simulink library "HelicopterBlockset"  (Simulink 5.0)
values from neighbouring files (symbols this model uses):
  alt_err_limit = 20    [DESIGNOR.M]    (also in HELICOPT.MAT)
  body_inertia = [0.8  0  0; 0  5  0; 0  0  5]    [HELICOPT.MAT]    (also in MODELPAR.M = body_mass *      [body_radius^2/2 0 0; 0 body_length^2/2 0; )
  body_mass = 10    [HELICOPT.MAT]    (also in MODELPAR.M)
  Cd = 0.1    [HELICOPT.MAT]    (also in MODELPAR.M)
  Cp = 0.10    (= 0.1)    [DESIGNOR.M]    (also in HELICOPT.MAT)
  Cq = 0.15    [DESIGNOR.M]    (also in HELICOPT.MAT)
  dt = 0.01    [HELICOPT.MAT]    (also in MODELPAR.M)
  Kd = 5    [DESIGNOR.M]    (also in HELICOPT.MAT)
  Kp = 0.8    [DESIGNOR.M]    (also in HELICOPT.MAT)
  mr_angle_ic = 90    [HELICOPT.MAT]    (also in MODELPAR.M)
  mr_inertia = [3.125e-05  0  0; 0  0.05  0; 0  0  0.05]    [HELICOPT.MAT]    (also in MODELPAR.M = mr_mass *      [mr_radius^2/2 0 0; 0 mr_length^2/2 0; 0 0 mr)
  mr_mass = 0.1    [HELICOPT.MAT]    (also in MODELPAR.M)
  mr_vel = -7161.97243914    [HELICOPT.MAT]    (also in MODELPAR.M)
  N = Nu + K*Nx    [SSDESIGN.M]
  N_p = 36.4154159163    [HELICOPT.MAT]
  N_r = -5.86917812224    [HELICOPT.MAT]
  N_v = 5.28688842277    [HELICOPT.MAT]
  N_y = -0.0302858280261    [HELICOPT.MAT]
  ssobsctrl_p =     [HELICOPT.MAT]
  ssobsctrl_r =     [HELICOPT.MAT]
  ssobsctrl_v =     [HELICOPT.MAT]
  ssobsctrl_y =     [HELICOPT.MAT]
  tau = 0.8    [DESIGNOR.M]    (also in HELICOPT.MAT)
  tilt_limit = 5    [DESIGNOR.M]    (also in HELICOPT.MAT)
  tr_inertia = [1.125e-06  0  0; 0  0.0008  0; 0  0  0.0008]    [HELICOPT.MAT]    (also in MODELPAR.M = tr_mass *      [tr_radius^2/2 0 0; 0 tr_length^2/2 0; 0 0 tr)
  tr_mass = 0.01    [HELICOPT.MAT]    (also in MODELPAR.M)
  tr_vel = 14323.9448783    [HELICOPT.MAT]    (also in MODELPAR.M)
  trim_lift_force = -99.1791    [HELICOPT.MAT]    (also in MODELPAR.M = -(body_mass + mr_mass + tr_mass) * gravity_vector(3))
  trim_pitch_mom = -0.04905    [HELICOPT.MAT]    (also in MODELPAR.M = (mr_mass*(mr_position(1) - body_position_ic(1)) +      tr_ma)
  waypoint = [-100 -100 0 0 -100 -100 -200 -200 -100 -100 -200 -200 ... (84 elements, 14x6)]    [HELICOPT.MAT]    (also in MODELPAR.M = [      100,   0,  25,  0,  0,  0;      100, 100,  25,  0,  0)
undefined symbols (not defined in the file or in its folder): Ad, Bd, Dd, dend, icd, numd
libraries: fixpt_lib_4 x19, mblibv1 x18, simulink x3, discretizing x1
settings Model: LastModifiedBy=Jim

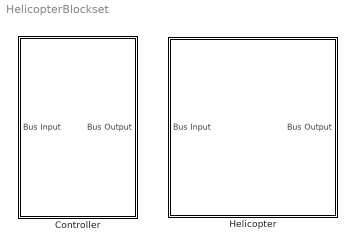
== system HelicopterBlockset ==
  Controller : Subsystem  TreatAsAtomicUnit=on
  Helicopter : Subsystem

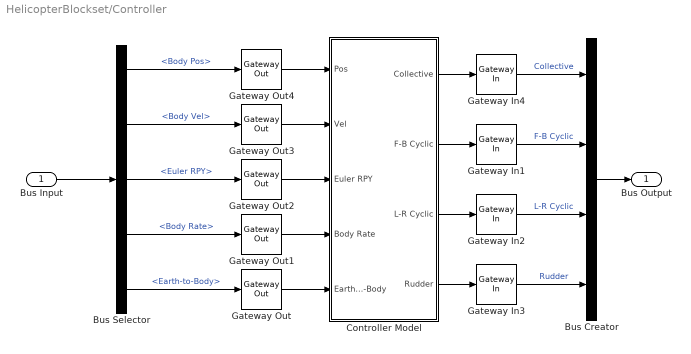
== system HelicopterBlockset/Controller ==
  Bus Input : Inport
  Bus Creator : BusCreator
  Bus Selector : BusSelector  OutputSignals=Body Pos,Body Vel,Euler RPY,Body Rate,Earth-to-Body
  Controller Model : Subsystem
  Gateway In{1..4} (4 alike) : fixpt_lib_4/Data Type/Gateway In  InRealWorld=Real World Value  OutputDataTypeScalingMode=Specify via dialog  OutDataType=sfix(16)  OutScaling=2^-8  RndMeth=Nearest  DoSatur=on
  Gateway Out{,1..4} (5 alike) : fixpt_lib_4/Data Type/Gateway Out  OutRealWorld=Real World Value  OutBuiltInType=double  RndMeth=Nearest  DoSatur=off
  Bus Output : Outport
  wires:
  Gateway In3/1 -> Bus Creator/4  "Rudder"
  Gateway In2/1 -> Bus Creator/3  "L-R Cyclic"
  Gateway In1/1 -> Bus Creator/2  "F-B Cyclic"
  Gateway In4/1 -> Bus Creator/1  "Collective"
  Gateway Out4/1 -> Controller Model/1(Pos)
  Gateway Out3/1 -> Controller Model/2(Vel)
  Gateway Out2/1 -> Controller Model/3(Euler RPY)
  Gateway Out1/1 -> Controller Model/4(Body Rate)
  Gateway Out/1 -> Controller Model/5(Earth-to-Body)
  Bus Input/1 -> Bus Selector/1
  Bus Creator/1 -> Bus Output/1
  Controller Model/4(Rudder) -> Gateway In3/1
  Bus Selector/2 -> Gateway Out3/1  "<Body Vel>"
  Controller Model/3(L-R Cyclic) -> Gateway In2/1
  Bus Selector/5 -> Gateway Out/1  "<Earth-to-Body>"
  Controller Model/2(F-B Cyclic) -> Gateway In1/1
  Controller Model/1(Collective) -> Gateway In4/1
  Bus Selector/4 -> Gateway Out1/1  "<Body Rate>"
  Bus Selector/3 -> Gateway Out2/1  "<Euler RPY>"
  Bus Selector/1 -> Gateway Out4/1  "<Body Pos>"

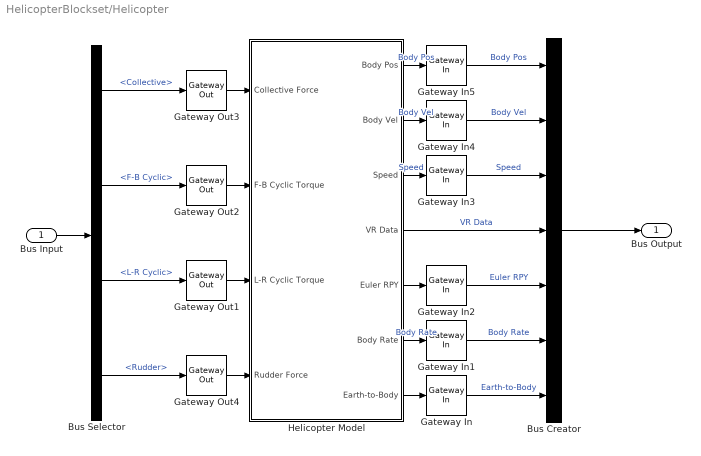
== system HelicopterBlockset/Helicopter ==
  Bus Input : Inport
  Bus Creator : BusCreator  Inputs=7
  Bus Selector : BusSelector  OutputSignals=Collective,F-B Cyclic,L-R Cyclic,Rudder
  Gateway In : fixpt_lib_4/Data Type/Gateway In  InRealWorld=Real World Value  OutputDataTypeScalingMode=Specify via dialog  OutDataType=sfix(8)  OutScaling=2^-7  RndMeth=Nearest  DoSatur=on
  Gateway In1 : fixpt_lib_4/Data Type/Gateway In  InRealWorld=Real World Value  OutputDataTypeScalingMode=Specify via dialog  OutDataType=sfix(16)  OutScaling=2^-7  RndMeth=Nearest  DoSatur=on
  Gateway In2 : fixpt_lib_4/Data Type/Gateway In  InRealWorld=Real World Value  OutputDataTypeScalingMode=Specify via dialog  OutDataType=sfix(16)  OutScaling=2^-7  RndMeth=Nearest  DoSatur=on
  Gateway In3 : fixpt_lib_4/Data Type/Gateway In  InRealWorld=Real World Value  OutputDataTypeScalingMode=Specify via dialog  OutDataType=sfix(16)  OutScaling=2^-8  RndMeth=Nearest  DoSatur=on
  Gateway In4 : fixpt_lib_4/Data Type/Gateway In  InRealWorld=Real World Value  OutputDataTypeScalingMode=Specify via dialog  OutDataType=sfix(16)  OutScaling=2^-8  RndMeth=Nearest  DoSatur=on
  Gateway In5 : fixpt_lib_4/Data Type/Gateway In  InRealWorld=Real World Value  OutputDataTypeScalingMode=Specify via dialog  OutDataType=sfix(32)  OutScaling=2^-4  RndMeth=Nearest  DoSatur=on
  Gateway Out{1..4} (4 alike) : fixpt_lib_4/Data Type/Gateway Out  OutRealWorld=Real World Value  OutBuiltInType=double  RndMeth=Nearest  DoSatur=off
  Helicopter Model : Subsystem
  Bus Output : Outport
  wires:
  Gateway Out3/1 -> Helicopter Model/1(Collective Force)
  Gateway Out2/1 -> Helicopter Model/2(F-B Cyclic Torque)
  Gateway Out1/1 -> Helicopter Model/3(L-R Cyclic Torque)
  Gateway Out4/1 -> Helicopter Model/4(Rudder Force)
  Gateway In5/1 -> Bus Creator/1  "Body Pos"
  Gateway In4/1 -> Bus Creator/2  "Body Vel"
  Gateway In3/1 -> Bus Creator/3  "Speed"
  Gateway In2/1 -> Bus Creator/5  "Euler RPY"
  Gateway In1/1 -> Bus Creator/6  "Body Rate"
  Gateway In/1 -> Bus Creator/7  "Earth-to-Body"
  Bus Creator/1 -> Bus Output/1
  Bus Input/1 -> Bus Selector/1
  Helicopter Model/7(Earth-to-Body) -> Gateway In/1
  Bus Selector/4 -> Gateway Out4/1  "<Rudder>"
  Helicopter Model/6(Body Rate) -> Gateway In1/1  "Body Rate"
  Helicopter Model/5(Euler RPY) -> Gateway In2/1
  Helicopter Model/4(VR Data) -> Bus Creator/4  "VR Data"
  Helicopter Model/3(Speed) -> Gateway In3/1  "Speed"
  Helicopter Model/2(Body Vel) -> Gateway In4/1  "Body Vel"
  Bus Selector/3 -> Gateway Out1/1  "<L-R Cyclic>"
  Helicopter Model/1(Body Pos) -> Gateway In5/1  "Body Pos"
  Bus Selector/2 -> Gateway Out2/1  "<F-B Cyclic>"
  Bus Selector/1 -> Gateway Out3/1  "<Collective>"

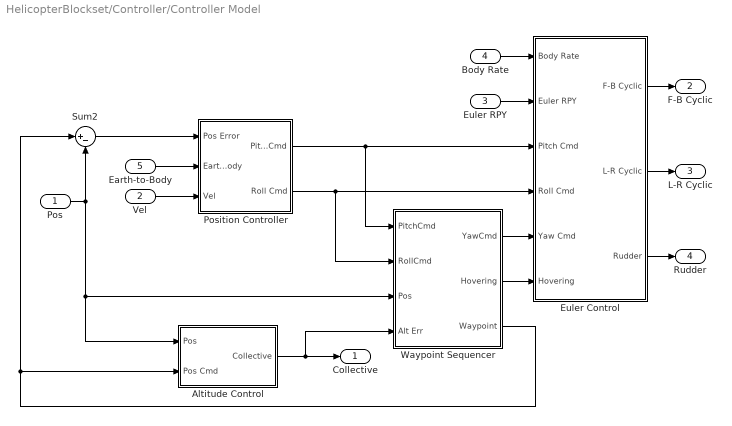
== system HelicopterBlockset/Controller/Controller Model ==
  Pos : Inport
  Vel : Inport  Port=2
  Euler RPY : Inport  Port=3
  Body Rate : Inport  Port=4
  Earth-to-Body : Inport  Port=5
  Altitude Control : Subsystem
  Euler Control : Subsystem
  Position Controller : Subsystem
  Sum2 : Sum  Inputs=|+-  SaturateOnIntegerOverflow=on
  Waypoint Sequencer : Subsystem
  Collective : Outport
  F-B Cyclic : Outport  Port=2
  L-R Cyclic : Outport  Port=3
  Rudder : Outport  Port=4
  wires:
  Waypoint Sequencer/2(Hovering) -> Euler Control/6(Hovering)
  Earth-to-Body/1 -> Position Controller/2(Earth-to-Body)
  Euler Control/3(Rudder) -> Rudder/1
  Euler Control/2(L-R Cyclic) -> L-R Cyclic/1
  Euler Control/1(F-B Cyclic) -> F-B Cyclic/1
  Euler RPY/1 -> Euler Control/2(Euler RPY)
  Body Rate/1 -> Euler Control/1(Body Rate)
  Altitude Control/1(Collective) -> Collective/1, Waypoint Sequencer/4(Alt Err)
  Vel/1 -> Position Controller/3(Vel)
  Waypoint Sequencer/1(YawCmd) -> Euler Control/5(Yaw Cmd)
  Pos/1 -> Sum2/2, Waypoint Sequencer/3(Pos), Altitude Control/1(Pos)
  Sum2/1 -> Position Controller/1(Pos Error)
  Position Controller/2(Roll Cmd) -> Euler Control/4(Roll Cmd), Waypoint Sequencer/2(RollCmd)
  Position Controller/1(Pitch Cmd) -> Euler Control/3(Pitch Cmd), Waypoint Sequencer/1(PitchCmd)
  Waypoint Sequencer/3(Waypoint) -> Altitude Control/2(Pos Cmd), Sum2/1

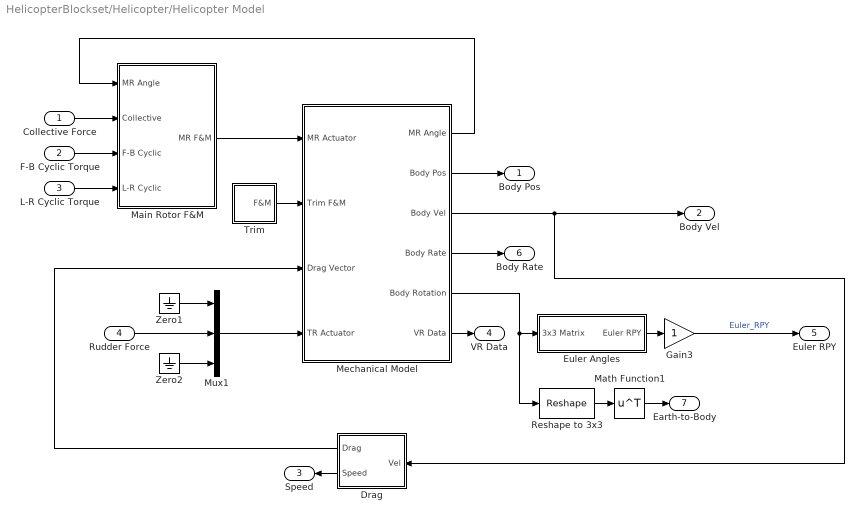
== system HelicopterBlockset/Helicopter/Helicopter Model ==
  Collective Force : Inport
  F-B Cyclic Torque : Inport  Port=2
  L-R Cyclic Torque : Inport  Port=3
  Rudder Force : Inport  Port=4
  Drag : Subsystem  Orientation=left
  Euler Angles : Subsystem
  Gain3 : Gain  SaturateOnIntegerOverflow=on
  Main Rotor F&M : Subsystem
  Math Function1 : Math  Operator=transpose
  Mechanical Model : Subsystem
  Mux1 : Mux  Inputs=3
  Reshape to 3x3 : simulink/Math Operations/Reshape  OutputDimensionality=Customize  OutputDimensions=[3,3]
  Trim : Subsystem
  Zero1 : Ground
  Zero2 : Ground
  Body Pos : Outport
  Body Vel : Outport  Port=2
  Speed : Outport  Orientation=left  Port=3
  VR Data : Outport  Port=4
  Euler RPY : Outport  Port=5  InitialOutput=0
  Body Rate : Outport  Port=6
  Earth-to-Body : Outport  Port=7  InitialOutput=0
  wires:
  Gain3/1 -> Euler RPY/1  "Euler_RPY"
  Drag/2(Speed) -> Speed/1
  Mechanical Model/6(VR Data) -> VR Data/1
  Mechanical Model/2(Body Pos) -> Body Pos/1
  Mechanical Model/3(Body Vel) -> Body Vel/1, Drag/1(Vel)
  Main Rotor F&M/1(MR F&M) -> Mechanical Model/1(MR Actuator)
  Mux1/1 -> Mechanical Model/4(TR Actuator)
  Zero1/1 -> Mux1/1
  Euler Angles/1(Euler RPY) -> Gain3/1
  L-R Cyclic Torque/1 -> Main Rotor F&M/4(L-R Cyclic)
  F-B Cyclic Torque/1 -> Main Rotor F&M/3(F-B Cyclic)
  Rudder Force/1 -> Mux1/2
  Collective Force/1 -> Main Rotor F&M/2(Collective)
  Trim/1(F&M) -> Mechanical Model/2(Trim F&M)
  Mechanical Model/4(Body Rate) -> Body Rate/1
  Mechanical Model/5(Body Rotation) -> Euler Angles/1(3x3 Matrix), Reshape to 3x3/1
  Reshape to 3x3/1 -> Math Function1/1
  Math Function1/1 -> Earth-to-Body/1
  Mechanical Model/1(MR Angle) -> Main Rotor F&M/1(MR Angle)
  Zero2/1 -> Mux1/3
  Drag/1(Drag) -> Mechanical Model/3(Drag Vector)

== system HelicopterBlockset/Controller/Controller Model/Altitude Control ==
  Pos : Inport
  Pos Cmd : Inport  Port=2
  Alt Limit : Saturate  UpperLimit=alt_err_limit  LowerLimit=-alt_err_limit
  Altitude Controller : Subsystem
  Demux1 : Demux  Outputs=3
  Demux2 : Demux  Outputs=3
  Terminator{2..3,5..6} (4 alike) : Terminator
  Collective : Outport
  wires:
  Alt Limit/1 -> Collective/1
  Pos Cmd/1 -> Demux1/1
  Pos/1 -> Demux2/1
  Altitude Controller/1(u) -> Alt Limit/1
  Demux2/2 -> Terminator6/1
  Demux2/1 -> Terminator5/1
  Demux2/3 -> Altitude Controller/2(y)
  Demux1/3 -> Altitude Controller/1(r)
  Demux1/1 -> Terminator3/1
  Demux1/2 -> Terminator2/1

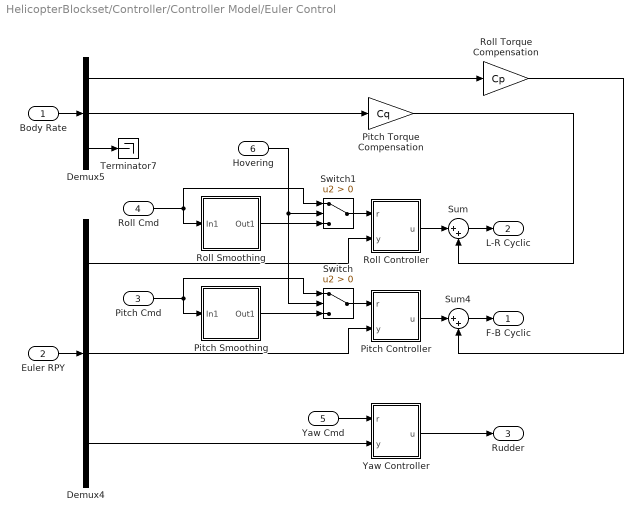
== system HelicopterBlockset/Controller/Controller Model/Euler Control ==
  Body Rate : Inport
  Euler RPY : Inport  Port=2
  Pitch Cmd : Inport  Port=3
  Roll Cmd : Inport  Port=4
  Yaw Cmd : Inport  Port=5
  Hovering : Inport  Port=6
  Demux4 : Demux  Outputs=3
  Demux5 : Demux  Outputs=3
  Pitch Controller : Subsystem
  Pitch Smoothing : Subsystem  mask(DiscretizedTransferFcn){Numerator=[1], Denominator=[tau 1], AbsTol=auto, SampleTime=dt, method=foh, Wc=1}
      mask prompts: Numerator "Numerator (enter in s-domain:)"; Denominator "Denominator (enter in s-domain:)"; AbsTol "Absolute tolerance:"; SampleTime "Sample time:"; Wc "Critical Frequency (Hz):"
      mask help: Continuous mask uses c2d to transform parameters onto the Discrete Transfer function block inside.
      mask init:
      | st=SampleTime;
      | if length(st)>1
      |     st=SampleTime(1);
      | end
      | if(st>0)
      |     [numd,dend] = sldiscutil('disctransferfcn',{st,method,Wc,Numerator,Denominator});
      | end	
      | s = get_param(gcb,'maskvalues');
      | nums = s{1};
      | dens = s{2};
      | %numc = eval(nums);
      | %denc = eval(dens);
      | sldiscutil('inittfmask', st);
      | if(st==0)
      | set_param([gcb '/Transfer Fcn'], 'AbsoluteTolerance', AbsTol);
      | end
      mask StyleString: edit,edit,edit,edit,popup(zoh|foh|tustin|prewarp|matched),edit
      mask CallbackString: ||||hidecrit|
      mask Display:
      | dpoly(nums,dens)
      | text( 0.5, 1.0, method, 'verticalAlignment','top')
  Pitch Torque Compensation : Gain  Gain=Cq  SaturateOnIntegerOverflow=on
  Roll Controller : Subsystem
  Roll Smoothing : Subsystem  mask(DiscretizedTransferFcn){Numerator=[1], Denominator=[tau 1], AbsTol=auto, SampleTime=dt, method=foh, Wc=1}
      mask prompts: Numerator "Numerator (enter in s-domain:)"; Denominator "Denominator (enter in s-domain:)"; AbsTol "Absolute tolerance:"; SampleTime "Sample time:"; Wc "Critical Frequency (Hz):"
      mask help: Continuous mask uses c2d to transform parameters onto the Discrete Transfer function block inside.
      mask init: same as HelicopterBlockset/Controller/Controller Model/Euler Control/Pitch Smoothing
      mask StyleString: edit,edit,edit,edit,popup(zoh|foh|tustin|prewarp|matched),edit
      mask CallbackString: ||||hidecrit|
      mask Display:
      | dpoly(nums,dens)
      | text( 0.5, 1.0, method, 'verticalAlignment','top')
  Roll Torque Compensation : Gain  Gain=Cp  SaturateOnIntegerOverflow=on
  Sum : Sum  Inputs=|++  SaturateOnIntegerOverflow=on
  Sum4 : Sum  Inputs=|++  SaturateOnIntegerOverflow=on
  Switch : Switch  Criteria=u2 > Threshold  SaturateOnIntegerOverflow=on
  Switch1 : Switch  Criteria=u2 > Threshold  SaturateOnIntegerOverflow=on
  Terminator7 : Terminator
  Yaw Controller : Subsystem
  F-B Cyclic : Outport
  L-R Cyclic : Outport  Port=2
  Rudder : Outport  Port=3
  wires:
  Roll Cmd/1 -> Switch1/1, Roll Smoothing/1(In1)
  Roll Smoothing/1(Out1) -> Switch1/3
  Pitch Smoothing/1(Out1) -> Switch/3
  Hovering/1 -> Switch/2, Switch1/2
  Switch1/1 -> Roll Controller/1(r)
  Pitch Cmd/1 -> Switch/1, Pitch Smoothing/1(In1)
  Switch/1 -> Pitch Controller/1(r)
  Yaw Controller/1(u) -> Rudder/1
  Yaw Cmd/1 -> Yaw Controller/1(r)
  Sum/1 -> L-R Cyclic/1
  Sum4/1 -> F-B Cyclic/1
  Euler RPY/1 -> Demux4/1
  Body Rate/1 -> Demux5/1
  Roll Controller/1(u) -> Sum/1
  Pitch Controller/1(u) -> Sum4/1
  Roll Torque Compensation/1 -> Sum4/2
  Demux5/1 -> Roll Torque Compensation/1
  Pitch Torque Compensation/1 -> Sum/2
  Demux5/2 -> Pitch Torque Compensation/1
  Demux5/3 -> Terminator7/1
  Demux4/3 -> Yaw Controller/2(y)
  Demux4/1 -> Roll Controller/2(y)
  Demux4/2 -> Pitch Controller/2(y)

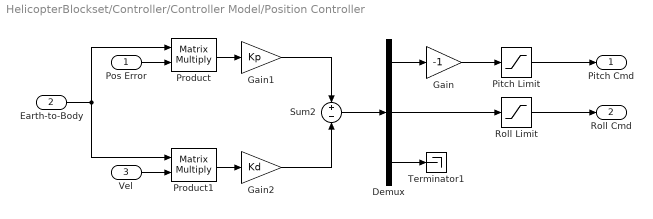
== system HelicopterBlockset/Controller/Controller Model/Position Controller ==
  Pos Error : Inport
  Earth-to-Body : Inport  Port=2
  Vel : Inport  Port=3
  Demux : Demux  Outputs=3
  Gain : Gain  Gain=-1  SaturateOnIntegerOverflow=on
  Gain1 : Gain  Gain=Kp  SaturateOnIntegerOverflow=on
  Gain2 : Gain  Gain=Kd  SaturateOnIntegerOverflow=on
  Pitch Limit : Saturate  UpperLimit=tilt_limit  LowerLimit=-tilt_limit
  Product : Product  Multiplication=Matrix(*)  SaturateOnIntegerOverflow=on
  Product1 : Product  Multiplication=Matrix(*)  SaturateOnIntegerOverflow=on
  Roll Limit : Saturate  UpperLimit=tilt_limit  LowerLimit=-tilt_limit
  Sum2 : Sum  Inputs=+|-  SaturateOnIntegerOverflow=on
  Terminator1 : Terminator
  Pitch Cmd : Outport
  Roll Cmd : Outport  Port=2
  wires:
  Roll Limit/1 -> Roll Cmd/1
  Pitch Limit/1 -> Pitch Cmd/1
  Gain/1 -> Pitch Limit/1
  Demux/1 -> Gain/1
  Demux/2 -> Roll Limit/1
  Sum2/1 -> Demux/1
  Gain2/1 -> Sum2/2
  Gain1/1 -> Sum2/1
  Vel/1 -> Product1/2
  Pos Error/1 -> Product/2
  Product1/1 -> Gain2/1
  Earth-to-Body/1 -> Product/1, Product1/1
  Product/1 -> Gain1/1
  Demux/3 -> Terminator1/1

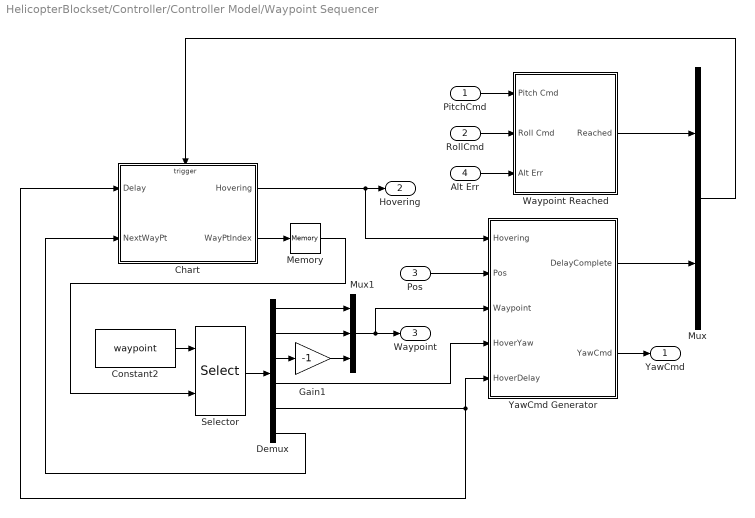
== system HelicopterBlockset/Controller/Controller Model/Waypoint Sequencer ==
  PitchCmd : Inport
  RollCmd : Inport  Port=2
  Pos : Inport  Port=3
  Alt Err : Inport  Port=4
  Chart : Stateflow chart
  Constant2 : Constant  Value=waypoint
  Demux : Demux  Outputs=6
  Gain1 : Gain  Gain=-1  SaturateOnIntegerOverflow=on
  Memory : Memory  X0=1
  Mux : Mux  Inputs=2
  Mux1 : Mux  Inputs=3
  Selector : Selector  InputType=Matrix  Elements=[1 3]  RowSrc=External  Columns=-1  InputPortWidth=3
  Waypoint Reached : Subsystem
  YawCmd Generator : Subsystem
  YawCmd : Outport
  Hovering : Outport  Port=2
  Waypoint : Outport  Port=3
  wires:
  Demux/6 -> Chart/2(NextWayPt)
  Chart/1(Hovering) -> Hovering/1, YawCmd Generator/1(Hovering)
  Gain1/1 -> Mux1/3
  Demux/3 -> Gain1/1
  Demux/2 -> Mux1/2
  Demux/1 -> Mux1/1
  Demux/4 -> YawCmd Generator/4(HoverYaw)
  Demux/5 -> Chart/1(Delay), YawCmd Generator/5(HoverDelay)
  YawCmd Generator/1(DelayComplete) -> Mux/2
  Memory/1 -> Selector/2
  YawCmd Generator/2(YawCmd) -> YawCmd/1
  Pos/1 -> YawCmd Generator/2(Pos)
  Chart/2(WayPtIndex) -> Memory/1
  Mux1/1 -> YawCmd Generator/3(Waypoint), Waypoint/1
  Mux/1 -> Chart/Trigger
  Waypoint Reached/1(Reached) -> Mux/1
  Constant2/1 -> Selector/1
  Selector/1 -> Demux/1
  Alt Err/1 -> Waypoint Reached/3(Alt Err)
  RollCmd/1 -> Waypoint Reached/2(Roll Cmd)
  PitchCmd/1 -> Waypoint Reached/1(Pitch Cmd)

== system HelicopterBlockset/Helicopter/Helicopter Model/Drag ==
  Vel : Inport
  Constant2 : Constant  Value=-Cd
  Dot Product : simulink/Math Operations/Dot Product
  Gain1 : Gain  SaturateOnIntegerOverflow=on
  Math Function : Math  Operator=sqrt
  Product2 : Product  Inputs=3  SaturateOnIntegerOverflow=on
  Drag : Outport
  Speed : Outport  Port=2
  wires:
  Gain1/1 -> Speed/1  "Speed"
  Dot Product/1 -> Math Function/1
  Math Function/1 -> Gain1/1, Product2/3
  Constant2/1 -> Product2/1
  Product2/1 -> Drag/1
  Vel/1 -> Dot Product/1, Dot Product/2, Product2/2

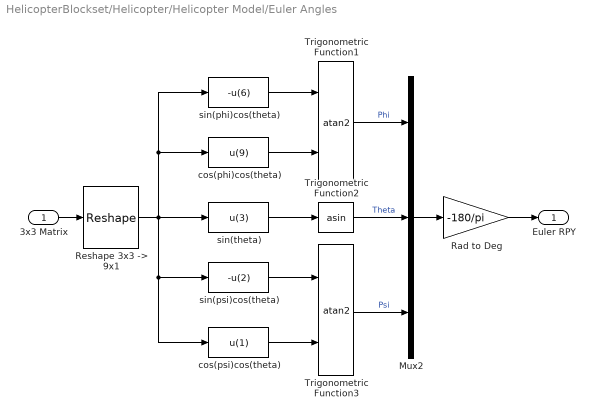
== system HelicopterBlockset/Helicopter/Helicopter Model/Euler Angles ==
  3x3 Matrix : Inport
  Mux2 : Mux  Inputs=3
  Rad to Deg : Gain  Gain=-180/pi  SaturateOnIntegerOverflow=on
  "Reshape 3x3 -> 9x1" : simulink/Math Operations/Reshape  OutputDimensionality=Column vector  OutputDimensions=[1,1]
  Trigonometric Function1 : Trigonometry  Operator=atan2
  Trigonometric Function2 : Trigonometry  Operator=asin
  Trigonometric Function3 : Trigonometry  Operator=atan2
  cos(phi)cos(theta) : Fcn  Expr=u(9)
  cos(psi)cos(theta) : Fcn  Expr=u(1)
  sin(phi)cos(theta) : Fcn  Expr=-u(6)
  sin(psi)cos(theta) : Fcn  Expr=-u(2)
  sin(theta) : Fcn  Expr=u(3)
  Euler RPY : Outport  InitialOutput=0
  wires:
  3x3 Matrix/1 -> "Reshape 3x3 -> 9x1"/1
  sin(theta)/1 -> Trigonometric Function2/1
  sin(phi)cos(theta)/1 -> Trigonometric Function1/1
  cos(phi)cos(theta)/1 -> Trigonometric Function1/2
  sin(psi)cos(theta)/1 -> Trigonometric Function3/1
  cos(psi)cos(theta)/1 -> Trigonometric Function3/2
  Trigonometric Function1/1 -> Mux2/1  "Phi"
  Trigonometric Function2/1 -> Mux2/2  "Theta"
  Trigonometric Function3/1 -> Mux2/3  "Psi"
  Mux2/1 -> Rad to Deg/1
  "Reshape 3x3 -> 9x1"/1 -> sin(theta)/1, sin(phi)cos(theta)/1, cos(phi)cos(theta)/1, sin(psi)cos(theta)/1, cos(psi)cos(theta)/1
  Rad to Deg/1 -> Euler RPY/1

== system HelicopterBlockset/Helicopter/Helicopter Model/Main Rotor F&M ==
  MR Angle : Inport
  Collective : Inport  Port=2
  F-B Cyclic : Inport  Port=3
  L-R Cyclic : Inport  Port=4
  Cosine of Blade Angle : Trigonometry  Operator=cos
  Mux : Mux  Inputs=6
  Product : Product  SaturateOnIntegerOverflow=on
  Product1 : Product  SaturateOnIntegerOverflow=on
  Sine of Blade Angle : Trigonometry
  Sum : Sum  Inputs=|++  SaturateOnIntegerOverflow=on
  Zero : Ground
  Zero1 : Ground
  MR F&M : Outport
  wires:
  MR Angle/1 -> Sine of Blade Angle/1, Cosine of Blade Angle/1
  Sine of Blade Angle/1 -> Product1/1
  Product1/1 -> Sum/2
  Product/1 -> Sum/1
  Cosine of Blade Angle/1 -> Product/1
  Sum/1 -> Mux/2
  Mux/1 -> MR F&M/1
  F-B Cyclic/1 -> Product/2
  L-R Cyclic/1 -> Product1/2
  Zero1/1 -> Mux/3, Mux/5, Mux/4
  Collective/1 -> Mux/6
  Zero/1 -> Mux/1

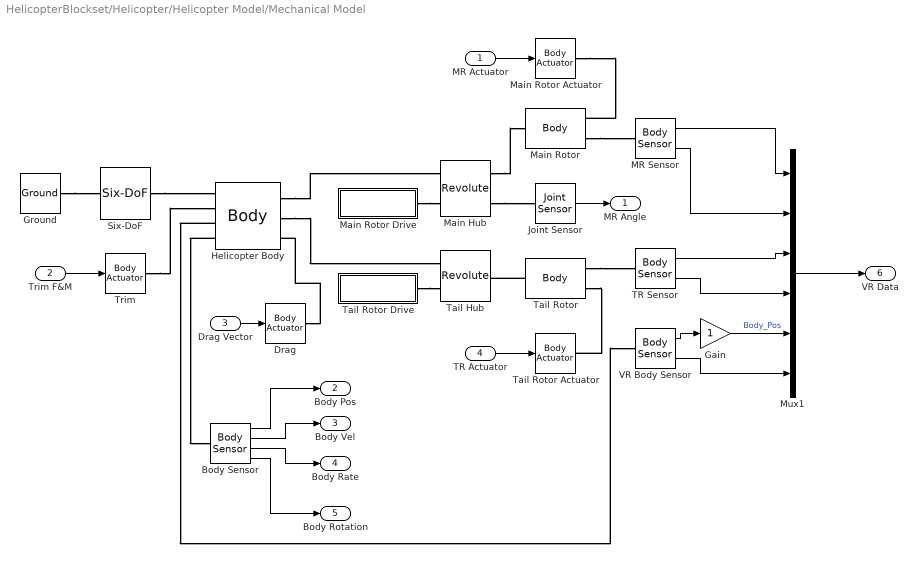
== system HelicopterBlockset/Helicopter/Helicopter Model/Mechanical Model ==
  MR Actuator : Inport
  Trim F&M : Inport  Port=2
  Drag Vector : Inport  Port=3
  TR Actuator : Inport  Port=4
  Body Sensor : mblibv1/Sensors &  Actuators/Body Sensor  Tag=__orphan__  PortType=blob  PhysicalDomain=Mechanical  Muxed=off  Pose=on  Angle=on  AngleUnits=deg  ArcVelocity=on  ArcVelocityUnits=deg/s  ArcAcceleration=off  ArcAccelerationUnits=deg/s^2  CoordPosition=on  CoordPositionUnits=m  Velocity=on  VelocityUnits=m/s  Acceleration=off  AccelerationUnits=m/s^2  Quaternion=on  QuaternionDT=off  QuaternionDDT=off  QuaternionUnits=off  OutputVector=[ 3 3 3 9 ]  IOID=sim_mech_taga8271b5312325fb6  ActiveIO=off  Width=18  DialogClass=MechanicalSensorBlock  ReferenceFrame=Absolute (World)
  Drag : mblibv1/Sensors &  Actuators/Body Actuator  Tag=__orphan__  PortType=blob  PhysicalDomain=Mechanical  ActuationStyle=Force  AngleUnits=deg  ArcVelocityUnits=deg/s  ArcAccelerationUnits=deg/s^2  CoordPositionUnits=m  VelocityUnits=m/s  AccelerationUnits=m/s^2  ForceUnits=N  TorqueUnits=N-m  IOID=sim_mech_tag546f64686babd5e8  ActiveIO=off  Width=3  DialogClass=MechanicalActuatorBlock  ReferenceFrame=Absolute (World)  Angle=off  CoordPosition=on  Force=on  Torque=off
  Gain : Gain  SaturateOnIntegerOverflow=on
  Ground : mblibv1/Bodies/Ground  Tag=__orphan__  PortType=workingframe  PhysicalDomain=Mechanical  DialogClass=GroundBlock  CoordPosition=ground_position  CoordPositionUnits=m  StateVectorMgrId=-1  MachineId=[0 0]
  Helicopter Body : mblibv1/Bodies/Body  PhysicalDomain=mechanical  SubClassName=Unknown  PortType=workingframe  LConnTagsString=CS1|CS4|CS6|CG  RConnTagsString=CS2|CS3|CS5  DialogClass=MechanicalBodyBlock  Mass=body_mass  MassUnits=kg  InertiaUnits=kg*m^2  Inertia=body_inertia  Shape=Cylinder  ShapeDims=[1 1]  ShapeUnits=m  ShapeUse=false  Density=1  DensityUnits=kg/m^3  DensityUse=false  CG=Left$CG$body_position_ic$WORLD$WORLD$m$body_orientation_ic$Euler Z-Y-X$deg$WORLD$true  WorkingFrames=Left$CS1$[0 0 0]$CG$CG$m$[0 0 0]$Euler Z-Y-X$deg$CG$true#Right$CS2$mr_position$CG$CG$m$mr_orientation$Euler Z-Y-X$deg$CG$true#Right$CS3$tr_position$CG$CG$m$tr_orientation$Euler Z-Y-X$deg$CG$true#Left$CS4$[0 0 0]$CG$CG$m$[0 0 0]$Euler Z-Y-X$deg$CG$true#Right$CS5$[0 0 0]$CG$CG$m$[0 0 0]$Euler Z-Y-X$deg$WORLD$true#Left$CS6$[0 0 0]$WORLD$WORLD$m$[0 0 0]$Euler Z-Y-X$deg$WORLD$true
  Joint Sensor : mblibv1/Sensors &  Actuators/Joint Sensor  Tag=__orphan__  PortType=blob  PhysicalDomain=Mechanical  Muxed=on  Pose=off  Angle=on  AngleUnits=rad  ArcVelocity=off  ArcVelocityUnits=deg/s  ArcAcceleration=off  ArcAccelerationUnits=deg/s^2  CoordPosition=on  CoordPositionUnits=m  Velocity=off  VelocityUnits=m/s  Acceleration=off  AccelerationUnits=m/s^2  Quaternion=on  QuaternionDT=off  QuaternionDDT=off  QuaternionUnits=off  OutputVector=[ 1 ]  IOID=sim_mech_tag96aebed2dbdd8e86  ActiveIO=off  Width=1  DialogClass=MechanicalSensorBlock  Primitive=R1  Force=off  ForceUnits=N  Torque=off  TorqueUnits=N-m  ReferenceFrame=Absolute (INERTIAL)  ReactionSensedSide=Base  ReactionReferenceFrame=Absolute (World)  ReactionForce=off  ReactionForceUnits=N  ReactionMoment=off  ReactionMomentUnits=N-m
  MR Sensor : mblibv1/Sensors &  Actuators/Body Sensor  Tag=__orphan__  PortType=blob  PhysicalDomain=Mechanical  Muxed=off  Pose=on  Angle=on  AngleUnits=deg  ArcVelocity=off  ArcVelocityUnits=deg/s  ArcAcceleration=off  ArcAccelerationUnits=deg/s^2  CoordPosition=on  CoordPositionUnits=m  Velocity=off  VelocityUnits=m/s  Acceleration=off  AccelerationUnits=m/s^2  Quaternion=on  QuaternionDT=off  QuaternionDDT=off  QuaternionUnits=off  OutputVector=[ 3 9 ]  IOID=sim_mech_tag28ea6e92d6f2dcb9  ActiveIO=off  Width=12  DialogClass=MechanicalSensorBlock  ReferenceFrame=Absolute (World)
  Main Hub : mblibv1/Joints/Revolute  PhysicalDomain=mechanical  SubClassName=Unknown  PortType=blob  LConnTagsString=__newl0|SA1  RConnTagsString=__newr0|SA1  NumSAPorts=2  CutJoint=off  MarkAsCut=off  Primitives=revolute  PrimitiveProps=R1$Base$mr_rotation_axis$revolute  DialogClass=JointBlock
  Main Rotor : mblibv1/Bodies/Body  PhysicalDomain=mechanical  SubClassName=Unknown  PortType=workingframe  LConnTagsString=CG  RConnTagsString=CS1|CS2  DialogClass=MechanicalBodyBlock  Mass=mr_mass  MassUnits=kg  InertiaUnits=kg*m^2  Inertia=mr_inertia  Shape=Cylinder  ShapeDims=[1 1]  ShapeUnits=m  ShapeUse=false  Density=1  DensityUnits=kg/m^3  DensityUse=false  CG=Left$CG$[0 0 0]$ADJOINING$ADJOINING$m$[0 0 0]$Euler Z-Y-X$deg$ADJOINING$true  WorkingFrames=Right$CS1$[0 0 0]$CG$CG$m$[0 0 0]$Euler Z-Y-X$deg$CG$true#Right$CS2$[0 0 0]$CG$CG$m$[0 0 0]$Euler Z-Y-X$deg$CG$true
  Main Rotor Actuator : mblibv1/Sensors &  Actuators/Body Actuator  Tag=__orphan__  PortType=blob  PhysicalDomain=Mechanical  ActuationStyle=Force  AngleUnits=deg  ArcVelocityUnits=deg/s  ArcAccelerationUnits=deg/s^2  CoordPositionUnits=m  VelocityUnits=m/s  AccelerationUnits=m/s^2  ForceUnits=N  TorqueUnits=N-m  IOID=sim_mech_tagaedf08eea5f3a52c  ActiveIO=off  Width=6  DialogClass=MechanicalActuatorBlock  ReferenceFrame=Local (Body CS)  Angle=off  CoordPosition=on  Force=on  Torque=on
  Main Rotor Drive : Subsystem
  Mux1 : Mux  Inputs=6
  Six-DoF : mblibv1/Joints/Six-DoF  PhysicalDomain=mechanical  SubClassName=Unknown  PortType=blob  LConnTagsString=__newl0  RConnTagsString=__newr0  NumSAPorts=0  CutJoint=off  MarkAsCut=off  Primitives=prismatic_prismatic_prismatic_spherical  PrimitiveProps=P1$WORLD$[1 0 0]$prismatic#P2$WORLD$[0 1 0]$prismatic#P3$WORLD$[0 0 1]$prismatic#S$WORLD$[0 0 0]$spherical  DialogClass=JointBlock
  TR Sensor : mblibv1/Sensors &  Actuators/Body Sensor  Tag=__orphan__  PortType=blob  PhysicalDomain=Mechanical  Muxed=off  Pose=on  Angle=on  AngleUnits=deg  ArcVelocity=off  ArcVelocityUnits=deg/s  ArcAcceleration=off  ArcAccelerationUnits=deg/s^2  CoordPosition=on  CoordPositionUnits=m  Velocity=off  VelocityUnits=m/s  Acceleration=off  AccelerationUnits=m/s^2  Quaternion=on  QuaternionDT=off  QuaternionDDT=off  QuaternionUnits=off  OutputVector=[ 3 9 ]  IOID=sim_mech_tag28899ab8cbe27b35  ActiveIO=off  Width=12  DialogClass=MechanicalSensorBlock  ReferenceFrame=Absolute (World)
  Tail Hub : mblibv1/Joints/Revolute  PhysicalDomain=mechanical  SubClassName=Unknown  PortType=blob  LConnTagsString=__newl0|SA1  RConnTagsString=__newr0  NumSAPorts=1  CutJoint=off  MarkAsCut=off  Primitives=revolute  PrimitiveProps=R1$Base$tr_rotation_axis$revolute  DialogClass=JointBlock
  Tail Rotor : mblibv1/Bodies/Body  PhysicalDomain=mechanical  SubClassName=Unknown  PortType=workingframe  LConnTagsString=CG  RConnTagsString=CS1|CS2  DialogClass=MechanicalBodyBlock  Mass=tr_mass  MassUnits=kg  InertiaUnits=kg*m^2  Inertia=tr_inertia  Shape=Cylinder  ShapeDims=[1 1]  ShapeUnits=m  ShapeUse=false  Density=1  DensityUnits=kg/m^3  DensityUse=false  CG=Left$CG$[0 0 0]$ADJOINING$ADJOINING$m$[0 0 0]$Euler Z-Y-X$deg$ADJOINING$true  WorkingFrames=Right$CS1$[0 0 0]$CG$CG$m$[0 0 0]$Euler Z-Y-X$deg$CG$true#Right$CS2$[0 0 0]$CG$CG$m$[0 0 0]$Euler Z-Y-X$deg$CG$true
  Tail Rotor Actuator : mblibv1/Sensors &  Actuators/Body Actuator  Tag=__orphan__  PortType=blob  PhysicalDomain=Mechanical  ActuationStyle=Force  AngleUnits=deg  ArcVelocityUnits=deg/s  ArcAccelerationUnits=deg/s^2  CoordPositionUnits=m  VelocityUnits=m/s  AccelerationUnits=m/s^2  ForceUnits=N  TorqueUnits=N-m  IOID=sim_mech_tage47e8b5af151c66b  ActiveIO=off  Width=3  DialogClass=MechanicalActuatorBlock  ReferenceFrame=Local (Body CS)  Angle=off  CoordPosition=on  Force=on  Torque=off
  Tail Rotor Drive : Subsystem
  Trim : mblibv1/Sensors &  Actuators/Body Actuator  Tag=__orphan__  PortType=blob  PhysicalDomain=Mechanical  ActuationStyle=Force  AngleUnits=deg  ArcVelocityUnits=deg/s  ArcAccelerationUnits=deg/s^2  CoordPositionUnits=m  VelocityUnits=m/s  AccelerationUnits=m/s^2  ForceUnits=N  TorqueUnits=N-m  IOID=sim_mech_tag2c7a50e163fe73c2  ActiveIO=off  Width=6  DialogClass=MechanicalActuatorBlock  ReferenceFrame=Local (Body CS)  Angle=off  CoordPosition=on  Force=on  Torque=on
  VR Body Sensor : mblibv1/Sensors &  Actuators/Body Sensor  Tag=__orphan__  PortType=blob  PhysicalDomain=Mechanical  Muxed=off  Pose=on  Angle=on  AngleUnits=deg  ArcVelocity=off  ArcVelocityUnits=deg/s  ArcAcceleration=off  ArcAccelerationUnits=deg/s^2  CoordPosition=on  CoordPositionUnits=m  Velocity=off  VelocityUnits=m/s  Acceleration=off  AccelerationUnits=m/s^2  Quaternion=on  QuaternionDT=off  QuaternionDDT=off  QuaternionUnits=off  OutputVector=[ 3 9 ]  IOID=sim_mech_tag22680ff6817110c5  ActiveIO=off  Width=12  DialogClass=MechanicalSensorBlock  ReferenceFrame=Absolute (World)
  MR Angle : Outport
  Body Pos : Outport  Port=2
  Body Vel : Outport  Port=3
  Body Rate : Outport  Port=4
  Body Rotation : Outport  Port=5
  VR Data : Outport  Port=6
  wires:
  VR Body Sensor/1 -> Gain/1
  Gain/1 -> Mux1/5  "Body_Pos"
  Mux1/1 -> VR Data/1
  TR Sensor/2 -> Mux1/4
  TR Sensor/1 -> Mux1/3
  MR Sensor/2 -> Mux1/2
  MR Actuator/1 -> Main Rotor Actuator/1
  MR Sensor/1 -> Mux1/1
  Joint Sensor/1 -> MR Angle/1
  Trim F&M/1 -> Trim/1
  Body Sensor/1 -> Body Pos/1
  Body Sensor/2 -> Body Vel/1
  Body Sensor/3 -> Body Rate/1
  Body Sensor/4 -> Body Rotation/1
  Drag Vector/1 -> Drag/1
  TR Actuator/1 -> Tail Rotor Actuator/1
  VR Body Sensor/2 -> Mux1/6
  connections:
  Helicopter Body/LConn4 -- Body Sensor/LConn1
  Drag/RConn1 -- Helicopter Body/RConn3
  Ground/RConn1 -- Six-DoF/LConn1
  Six-DoF/RConn1 -- Helicopter Body/LConn1
  Helicopter Body/RConn1 -- Main Hub/LConn1
  Helicopter Body/RConn2 -- Tail Hub/LConn1
  Main Hub/RConn2 -- Joint Sensor/LConn1
  Main Rotor/RConn2 -- MR Sensor/LConn1
  Main Hub/RConn1 -- Main Rotor/LConn1
  Main Rotor Actuator/RConn1 -- Main Rotor/RConn1
  Tail Rotor Drive/RConn1 -- Tail Hub/LConn2
  Main Rotor Drive/RConn1 -- Main Hub/LConn2
  Tail Rotor/LConn1 -- Tail Hub/RConn1
  Tail Rotor/RConn2 -- Tail Rotor Actuator/RConn1
  Tail Rotor/RConn1 -- TR Sensor/LConn1
  Trim/RConn1 -- Helicopter Body/LConn2
  Helicopter Body/LConn3 -- VR Body Sensor/LConn1

== system HelicopterBlockset/Helicopter/Helicopter Model/Trim ==
  Constant : Constant  Value=trim_lift_force
  Constant1 : Constant  Value=trim_pitch_mom
  Mux2 : Mux  Inputs=6
  Zero2 : Ground
  F&M : Outport
  wires:
  Zero2/1 -> Mux2/1, Mux2/4, Mux2/5, Mux2/3
  Constant1/1 -> Mux2/2
  Constant/1 -> Mux2/6
  Mux2/1 -> F&M/1

== system HelicopterBlockset/Controller/Controller Model/Altitude Control/Altitude Controller ==
  r : Inport
  y : Inport  Port=2
  Gain : Gain  Gain=N_v  SaturateOnIntegerOverflow=on
  Mux : Mux  Inputs=2
  Observer- Controller : Subsystem  mask(DiscretizedStateSpace){A=ssobsctrl_v.a, B=ssobsctrl_v.b, C=ssobsctrl_v.c, D=ssobsctrl_v.d, ic=0, AbsTol=auto, SampleTime=dt, method=zoh, Wc=1}
      mask prompts: A "A (enter in s-domain:)"; B "B (enter in s-domain:)"; C "C (enter in s-domain:)"; D "D (enter in s-domain:)"; ic "Initial conditions (enter in s-domain:)"; AbsTol "Absolute tolerance"; SampleTime "Sample time:"; Wc "Critical Frequency (Hz):"
      mask help: Continuous mask uses c2d to transform parameters onto the Discrete State-Space block inside.
      mask init:
      | st=SampleTime;
      | if length(st)>1
      |     st=SampleTime(1);
      | end
      | if(st>0)
      |     [Ad, Bd, Cd, Dd, icd] = sldiscutil('discstatespace', {st,method,Wc,A,B,C,D,ic});
      | end
      | sldiscutil('initssmask', st);
      | if(st==0)
      | set_param([gcb '/State Space'], 'AbsoluteTolerance', AbsTol);
      | end
      mask StyleString: edit,edit,edit,edit,edit,edit,edit,popup(zoh|foh|tustin|prewarp|matched),edit
      mask CallbackString: |||||||hidecrit|
      mask Display:
      | text( 0.5, 0.65, 'x'' = Ax+Bu', 'horizontalAlignment', 'center');
      | text( 0.5, 0.4, 'y = Cx+Du', 'horizontalAlignment', 'center');
      | text( 0.5, 1.0, method, 'verticalAlignment', 'top')
  Sum : Sum  Inputs=++|  SaturateOnIntegerOverflow=on
  u : Outport
  wires:
  y/1 -> Mux/1
  r/1 -> Gain/1
  Gain/1 -> Sum/1
  Observer- Controller/1(Out1) -> Sum/2
  Sum/1 -> Mux/2, u/1
  Mux/1 -> Observer- Controller/1(In1)

== system HelicopterBlockset/Controller/Controller Model/Euler Control/Pitch Controller ==
  r : Inport
  y : Inport  Port=2
  Gain : Gain  Gain=N_p  SaturateOnIntegerOverflow=on
  Mux : Mux  Inputs=2
  Observer- Controller : Subsystem  mask(DiscretizedStateSpace){A=ssobsctrl_p.a, B=ssobsctrl_p.b, C=ssobsctrl_p.c, D=ssobsctrl_p.d, ic=0, AbsTol=auto, SampleTime=dt, method=zoh, Wc=1}
      mask prompts: A "A (enter in s-domain:)"; B "B (enter in s-domain:)"; C "C (enter in s-domain:)"; D "D (enter in s-domain:)"; ic "Initial conditions (enter in s-domain:)"; AbsTol "Absolute tolerance"; SampleTime "Sample time:"; Wc "Critical Frequency (Hz):"
      mask help: Continuous mask uses c2d to transform parameters onto the Discrete State-Space block inside.
      mask init: same as HelicopterBlockset/Controller/Controller Model/Altitude Control/Altitude Controller/Observer- Controller
      mask StyleString: edit,edit,edit,edit,edit,edit,edit,popup(zoh|foh|tustin|prewarp|matched),edit
      mask CallbackString: |||||||hidecrit|
      mask Display:
      | text( 0.5, 0.65, 'x'' = Ax+Bu', 'horizontalAlignment', 'center');
      | text( 0.5, 0.4, 'y = Cx+Du', 'horizontalAlignment', 'center');
      | text( 0.5, 1.0, method, 'verticalAlignment', 'top')
  Sum : Sum  Inputs=++|  SaturateOnIntegerOverflow=on
  u : Outport
  wires:
  y/1 -> Mux/1
  r/1 -> Gain/1
  Gain/1 -> Sum/1
  Observer- Controller/1(Out1) -> Sum/2
  Sum/1 -> Mux/2, u/1
  Mux/1 -> Observer- Controller/1(In1)

== system HelicopterBlockset/Controller/Controller Model/Euler Control/Pitch Smoothing ==
  In1 : Inport
  Discrete Transfer Fcn : DiscreteTransferFcn  Numerator=numd  Denominator=dend  SampleTime=SampleTime
  Out1 : Outport
  wires:
  Discrete Transfer Fcn/1 -> Out1/1
  In1/1 -> Discrete Transfer Fcn/1

== system HelicopterBlockset/Controller/Controller Model/Euler Control/Roll Controller ==
  r : Inport
  y : Inport  Port=2
  Gain : Gain  Gain=N_r  SaturateOnIntegerOverflow=on
  Mux : Mux  Inputs=2
  Observer- Controller : Subsystem  mask(DiscretizedStateSpace){A=ssobsctrl_r.a, B=ssobsctrl_r.b, C=ssobsctrl_r.c, D=ssobsctrl_r.d, ic=0, AbsTol=auto, SampleTime=dt, method=zoh, Wc=1}
      mask prompts: A "A (enter in s-domain:)"; B "B (enter in s-domain:)"; C "C (enter in s-domain:)"; D "D (enter in s-domain:)"; ic "Initial conditions (enter in s-domain:)"; AbsTol "Absolute tolerance"; SampleTime "Sample time:"; Wc "Critical Frequency (Hz):"
      mask help: Continuous mask uses c2d to transform parameters onto the Discrete State-Space block inside.
      mask init: same as HelicopterBlockset/Controller/Controller Model/Altitude Control/Altitude Controller/Observer- Controller
      mask StyleString: edit,edit,edit,edit,edit,edit,edit,popup(zoh|foh|tustin|prewarp|matched),edit
      mask CallbackString: |||||||hidecrit|
      mask Display:
      | text( 0.5, 0.65, 'x'' = Ax+Bu', 'horizontalAlignment', 'center');
      | text( 0.5, 0.4, 'y = Cx+Du', 'horizontalAlignment', 'center');
      | text( 0.5, 1.0, method, 'verticalAlignment', 'top')
  Sum : Sum  Inputs=++|  SaturateOnIntegerOverflow=on
  u : Outport
  wires:
  y/1 -> Mux/1
  r/1 -> Gain/1
  Gain/1 -> Sum/1
  Observer- Controller/1(Out1) -> Sum/2
  Sum/1 -> Mux/2, u/1
  Mux/1 -> Observer- Controller/1(In1)

== system HelicopterBlockset/Controller/Controller Model/Euler Control/Roll Smoothing ==
  In1 : Inport
  Discrete Transfer Fcn : DiscreteTransferFcn  Numerator=numd  Denominator=dend  SampleTime=SampleTime
  Out1 : Outport
  wires:
  Discrete Transfer Fcn/1 -> Out1/1
  In1/1 -> Discrete Transfer Fcn/1

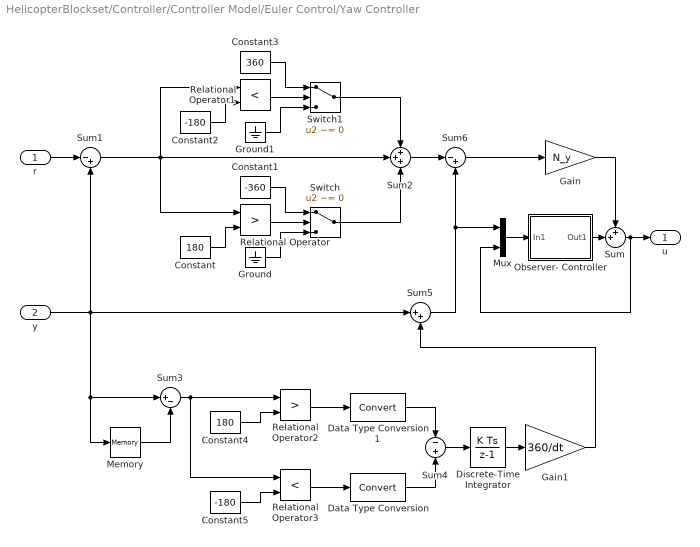
== system HelicopterBlockset/Controller/Controller Model/Euler Control/Yaw Controller ==
  r : Inport
  y : Inport  Port=2
  Constant : Constant  Value=180
  Constant1 : Constant  Value=-360
  Constant2 : Constant  Value=-180
  Constant3 : Constant  Value=360
  Constant4 : Constant  Value=180
  Constant5 : Constant  Value=-180
  Data Type Conversion : DataTypeConversion  SaturateOnIntegerOverflow=on
  Data Type Conversion1 : DataTypeConversion  SaturateOnIntegerOverflow=on
  Discrete-Time Integrator : DiscreteIntegrator  SampleTime=dt
  Gain : Gain  Gain=N_y  SaturateOnIntegerOverflow=on
  Gain1 : Gain  Gain=360/dt  SaturateOnIntegerOverflow=on
  Ground : Ground
  Ground1 : Ground
  Memory : Memory  X0=1
  Mux : Mux  Inputs=2
  Observer- Controller : Subsystem  mask(DiscretizedStateSpace){A=ssobsctrl_y.a, B=ssobsctrl_y.b, C=ssobsctrl_y.c, D=ssobsctrl_y.d, ic=0, AbsTol=auto, SampleTime=dt, method=zoh, Wc=1}
      mask prompts: A "A (enter in s-domain:)"; B "B (enter in s-domain:)"; C "C (enter in s-domain:)"; D "D (enter in s-domain:)"; ic "Initial conditions (enter in s-domain:)"; AbsTol "Absolute tolerance"; SampleTime "Sample time:"; Wc "Critical Frequency (Hz):"
      mask help: Continuous mask uses c2d to transform parameters onto the Discrete State-Space block inside.
      mask init: same as HelicopterBlockset/Controller/Controller Model/Altitude Control/Altitude Controller/Observer- Controller
      mask StyleString: edit,edit,edit,edit,edit,edit,edit,popup(zoh|foh|tustin|prewarp|matched),edit
      mask CallbackString: |||||||hidecrit|
      mask Display:
      | text( 0.5, 0.65, 'x'' = Ax+Bu', 'horizontalAlignment', 'center');
      | text( 0.5, 0.4, 'y = Cx+Du', 'horizontalAlignment', 'center');
      | text( 0.5, 1.0, method, 'verticalAlignment', 'top')
  Relational Operator : RelationalOperator  Operator=>
  Relational Operator1 : RelationalOperator  Operator=<
  Relational Operator2 : RelationalOperator  Operator=>
  Relational Operator3 : RelationalOperator  Operator=<
  Sum : Sum  Inputs=++|  SaturateOnIntegerOverflow=on
  Sum1 : Sum  Inputs=|-+  SaturateOnIntegerOverflow=on
  Sum2 : Sum  Inputs=+++  SaturateOnIntegerOverflow=on
  Sum3 : Sum  Inputs=|+-  SaturateOnIntegerOverflow=on
  Sum4 : Sum  Inputs=-|+  SaturateOnIntegerOverflow=on
  Sum5 : Sum  Inputs=|++  SaturateOnIntegerOverflow=on
  Sum6 : Sum  Inputs=|-+  SaturateOnIntegerOverflow=on
  Switch : Switch  Criteria=u2 ~= 0  Threshold=1  SaturateOnIntegerOverflow=on
  Switch1 : Switch  Criteria=u2 ~= 0  Threshold=1  SaturateOnIntegerOverflow=on
  u : Outport
  wires:
  Discrete-Time Integrator/1 -> Gain1/1
  Data Type Conversion/1 -> Sum4/2
  Data Type Conversion1/1 -> Sum4/1
  Sum5/1 -> Mux/1, Sum6/2
  Gain1/1 -> Sum5/2
  Sum4/1 -> Discrete-Time Integrator/1
  Relational Operator3/1 -> Data Type Conversion/1
  Constant5/1 -> Relational Operator3/2
  Relational Operator2/1 -> Data Type Conversion1/1
  Sum3/1 -> Relational Operator3/1, Relational Operator2/1
  Constant4/1 -> Relational Operator2/2
  Memory/1 -> Sum3/2
  Sum6/1 -> Gain/1
  Sum2/1 -> Sum6/1
  Switch1/1 -> Sum2/1
  Switch/1 -> Sum2/3
  Ground1/1 -> Switch1/3
  Constant3/1 -> Switch1/1
  Relational Operator1/1 -> Switch1/2
  Constant2/1 -> Relational Operator1/2
  Ground/1 -> Switch/3
  Constant1/1 -> Switch/1
  Relational Operator/1 -> Switch/2
  Constant/1 -> Relational Operator/2
  Sum1/1 -> Relational Operator1/1, Sum2/2, Relational Operator/1
  y/1 -> Sum3/1, Memory/1, Sum5/1, Sum1/2
  r/1 -> Sum1/1
  Gain/1 -> Sum/1
  Observer- Controller/1(Out1) -> Sum/2
  Sum/1 -> Mux/2, u/1
  Mux/1 -> Observer- Controller/1(In1)

== system HelicopterBlockset/Controller/Controller Model/Waypoint Sequencer/Waypoint Reached ==
  Pitch Cmd : Inport
  Roll Cmd : Inport  Port=2
  Alt Err : Inport  Port=3
  Abs : Abs  SaturateOnIntegerOverflow=on
  Abs1 : Abs  SaturateOnIntegerOverflow=on
  Abs2 : Abs  SaturateOnIntegerOverflow=on
  Constant : Constant  Value=tilt_limit
  Constant1 : Constant  Value=alt_err_limit
  Logical Operator : Logic  Inputs=3  AllPortsSameDT=off
  Sum : Sum  Inputs=-+|  SaturateOnIntegerOverflow=on
  Sum1 : Sum  Inputs=|+-  SaturateOnIntegerOverflow=on
  Sum2 : Sum  Inputs=|+-  SaturateOnIntegerOverflow=on
  Reached : Outport
  wires:
  Alt Err/1 -> Abs2/1
  Logical Operator/1 -> Reached/1
  Roll Cmd/1 -> Abs1/1
  Pitch Cmd/1 -> Abs/1
  Sum2/1 -> Logical Operator/3
  Constant1/1 -> Sum2/2
  Abs2/1 -> Sum2/1
  Sum/1 -> Logical Operator/2
  Sum1/1 -> Logical Operator/1
  Abs1/1 -> Sum/2
  Constant/1 -> Sum/1, Sum1/2
  Abs/1 -> Sum1/1

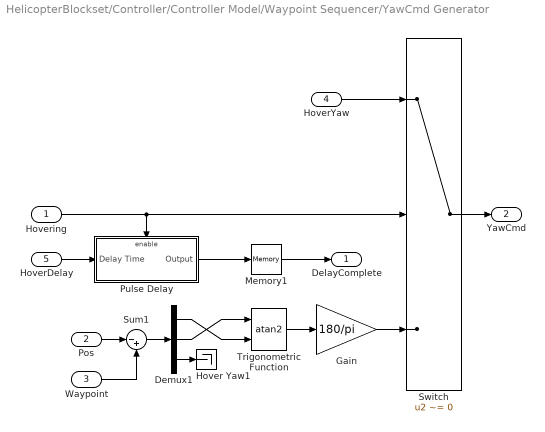
== system HelicopterBlockset/Controller/Controller Model/Waypoint Sequencer/YawCmd Generator ==
  Hovering : Inport
  Pos : Inport  Port=2
  Waypoint : Inport  Port=3
  HoverYaw : Inport  Port=4
  HoverDelay : Inport  Port=5
  Demux1 : Demux  Outputs=3
  Gain : Gain  Gain=180/pi  SaturateOnIntegerOverflow=on
  Hover Yaw1 : Terminator
  Memory1 : Memory  X0=1
  Pulse Delay : Subsystem  TreatAsAtomicUnit=on
  Sum1 : Sum  Inputs=|-+  SaturateOnIntegerOverflow=on
  Switch : Switch  Criteria=u2 ~= 0  SaturateOnIntegerOverflow=on
  Trigonometric Function : Trigonometry  Operator=atan2
  DelayComplete : Outport
  YawCmd : Outport  Port=2
  wires:
  Memory1/1 -> DelayComplete/1
  Demux1/1 -> Trigonometric Function/2
  Switch/1 -> YawCmd/1
  Pos/1 -> Sum1/1
  HoverYaw/1 -> Switch/1
  HoverDelay/1 -> Pulse Delay/1(Delay Time)
  Waypoint/1 -> Sum1/2
  Gain/1 -> Switch/3
  Trigonometric Function/1 -> Gain/1
  Sum1/1 -> Demux1/1
  Demux1/3 -> Hover Yaw1/1
  Demux1/2 -> Trigonometric Function/1
  Pulse Delay/1(Output) -> Memory1/1
  Hovering/1 -> Pulse Delay/Enable, Switch/2

== system HelicopterBlockset/Helicopter/Helicopter Model/Mechanical Model/Main Rotor Drive ==
  Constant : Constant  Value=0
  Integrator : Integrator  InitialCondition=mr_angle_ic
  Main Rotor Vel : Constant  Value=mr_vel
  Main Rotor Drive : mblibv1/Sensors &  Actuators/Joint Actuator  Tag=__orphan__  PortType=blob  PhysicalDomain=Mechanical  ActuationStyle=Motion  AngleUnits=deg  ArcVelocityUnits=deg/s  ArcAccelerationUnits=deg/s^2  CoordPositionUnits=m  VelocityUnits=m/s  AccelerationUnits=m/s^2  ForceUnits=N  TorqueUnits=N-m  IOID=sim_mech_tag31668bd053349131  ActiveIO=off  Width=3  DialogClass=MechanicalActuatorBlock  Primitive=R1  ReferenceFrame=Absolute (INERTIAL)
  Mux : Mux  Inputs=3
  Drive : PMIOPort  Orientation=left  Port=1  Side=right
  wires:
  Mux/1 -> Main Rotor Drive/1
  Main Rotor Vel/1 -> Integrator/1, Mux/2
  Integrator/1 -> Mux/1
  Constant/1 -> Mux/3
  connections:
  Drive/RConn1 -- Main Rotor Drive/RConn1

== system HelicopterBlockset/Helicopter/Helicopter Model/Mechanical Model/Tail Rotor Drive ==
  Constant : Constant  Value=0
  Integrator : Integrator  InitialCondition=mr_angle_ic
  Mux : Mux  Inputs=3
  Tail Rotor Vel : Constant  Value=tr_vel
  Tail Rotor Drive : mblibv1/Sensors &  Actuators/Joint Actuator  Tag=__orphan__  PortType=blob  PhysicalDomain=Mechanical  ActuationStyle=Motion  AngleUnits=deg  ArcVelocityUnits=deg/s  ArcAccelerationUnits=deg/s^2  CoordPositionUnits=m  VelocityUnits=m/s  AccelerationUnits=m/s^2  ForceUnits=N  TorqueUnits=N-m  IOID=sim_mech_tag917bda533aa8e98e  ActiveIO=off  Width=3  DialogClass=MechanicalActuatorBlock  Primitive=R1  ReferenceFrame=Absolute (INERTIAL)
  Drive : PMIOPort  Orientation=left  Port=1  Side=right
  wires:
  Mux/1 -> Tail Rotor Drive/1
  Integrator/1 -> Mux/1
  Constant/1 -> Mux/3
  Tail Rotor Vel/1 -> Mux/2, Integrator/1
  connections:
  Drive/RConn1 -- Tail Rotor Drive/RConn1

== system HelicopterBlockset/Controller/Controller Model/Altitude Control/Altitude Controller/Observer- Controller ==
  In1 : Inport
  Discrete State-Space : DiscreteStateSpace  A=Ad  B=Bd  C=Cd  D=Dd  X0=icd  SampleTime=SampleTime
  Out1 : Outport
  wires:
  In1/1 -> Discrete State-Space/1
  Discrete State-Space/1 -> Out1/1

== system HelicopterBlockset/Controller/Controller Model/Euler Control/Pitch Controller/Observer- Controller ==
  In1 : Inport
  Discrete State-Space : DiscreteStateSpace  A=Ad  B=Bd  C=Cd  D=Dd  X0=icd  SampleTime=SampleTime
  Out1 : Outport
  wires:
  In1/1 -> Discrete State-Space/1
  Discrete State-Space/1 -> Out1/1

== system HelicopterBlockset/Controller/Controller Model/Euler Control/Roll Controller/Observer- Controller ==
  In1 : Inport
  Discrete State-Space : DiscreteStateSpace  A=Ad  B=Bd  C=Cd  D=Dd  X0=icd  SampleTime=SampleTime
  Out1 : Outport
  wires:
  In1/1 -> Discrete State-Space/1
  Discrete State-Space/1 -> Out1/1

== system HelicopterBlockset/Controller/Controller Model/Euler Control/Yaw Controller/Observer- Controller ==
  In1 : Inport
  Discrete State-Space : DiscreteStateSpace  A=Ad  B=Bd  C=Cd  D=Dd  X0=icd  SampleTime=SampleTime
  Out1 : Outport
  wires:
  In1/1 -> Discrete State-Space/1
  Discrete State-Space/1 -> Out1/1

== system HelicopterBlockset/Controller/Controller Model/Waypoint Sequencer/YawCmd Generator/Pulse Delay ==
  note: Set the 'Delay Time' input to a value >= 0, then
      | 'Output' becomes true 'Delay Time' seconds after
      | the rising edge of the Enable input.
  Delay Time : Inport
  Enable : EnablePort  StatesWhenEnabling=reset
  Constant : Constant
  Discretized Transfer Fcn : discretizing/Discretized Transfer Fcn  Numerator=[1]  Denominator=[1 0]  AbsTol=auto  SampleTime=dt  method=foh  Wc=1
  Relational Operator : RelationalOperator
  Output : Outport
  wires:
  Delay Time/1 -> Relational Operator/2
  Relational Operator/1 -> Output/1
  Discretized Transfer Fcn/1 -> Relational Operator/1
  Constant/1 -> Discretized Transfer Fcn/1

== stateflow chart Controller/Controller Model/Waypoint Sequencer/Chart ==
  settings: updateMethod=DISCRETE  executeAtInitialization=1
  state Hover
    en: Hovering = 1;
    ex: Hovering = 0;
  state GuideToWayPt
  Hover -> (junction 6) : DelayComplete
  (default) -> GuideToWayPt
  GuideToWayPt -> (junction 5) : WayPtReached
  (junction 5) -> Hover : [Delay > 0]
  (junction 5) -> (junction 6)
  (junction 6) -> GuideToWayPt : / WayPtIndex = NextWayPt;
  (junction 6) -> GuideToWayPt : [NextWayPt == 0] / WayPtIndex++;
  data: Hovering output boolean; WayPtIndex output =1; Delay input; NextWayPt input
  events: WayPtReached input RISING_EDGE_EVENT; DelayComplete input RISING_EDGE_EVENT
